simulink library "controllerComponents"  (R2017b)
settings: Solver=VariableStepAuto  StartTime=0.0  StopTime=10.0  RelTol=1e-3
undefined symbols (not defined in the file): ctrl, env, plant
libraries: controllerComponents x14, simulink x3, lowLevel x3, vrlib x1, dspstat3 x1, dspsigops x1
settings Model: Creator=mitch  LastModifiedBy=mitch

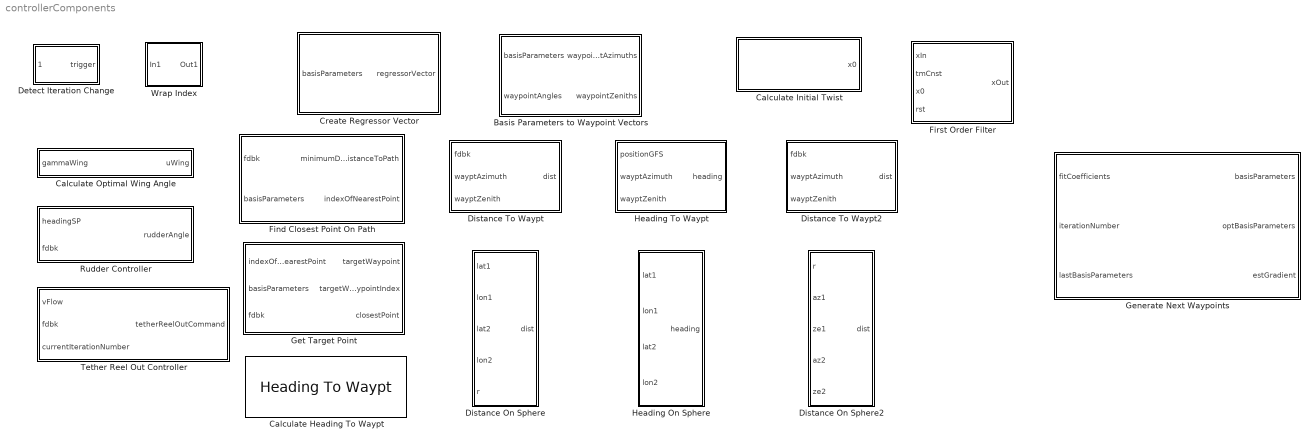
== system controllerComponents ==
  Basis Parameters to Waypoint Vectors : Subsystem
  Calculate Heading To Waypt : controllerComponents/Heading To Waypt
  Calculate Initial Twist : Subsystem
  Calculate Optimal Wing Angle : Subsystem
  Create Regressor Vector : Subsystem
  Detect Iteration Change : Subsystem
  Distance On Sphere : Subsystem
  Distance On Sphere2 : Subsystem
  Distance To Waypt : Subsystem
  Distance To Waypt2 : Subsystem
  Find Closest Point On Path : Subsystem
  First Order Filter : Subsystem
  Generate Next Waypoints : Subsystem
  Get Target Point : Subsystem
  Heading On Sphere : Subsystem
  Heading To Waypt : Subsystem
  Rudder Controller : Subsystem
  Tether Reel Out Controller : Subsystem
  Wrap Index : Subsystem

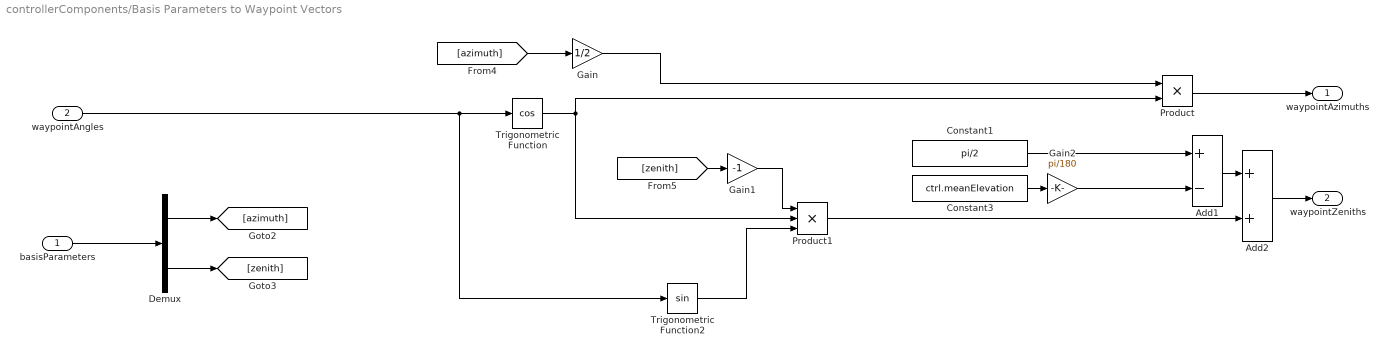
== system controllerComponents/Basis Parameters to Waypoint Vectors ==
  basisParameters : Inport
  waypointAngles : Inport  Port=2
  Add1 : Sum  Inputs=+-
  Add2 : Sum
  Constant1 : Constant  Value=pi/2
  Constant3 : Constant  Value=ctrl.meanElevation
  Demux : Demux  Outputs=2
  Gain : Gain  Gain=1/2
  Gain1 : Gain  Gain=-1
  Gain2 : Gain  Gain=pi/180
  Product : Product
  Product1 : Product  Inputs=3
  Trigonometric Function : Trigonometry  Operator=cos
  Trigonometric Function2 : Trigonometry
  waypointAzimuths : Outport
  waypointZeniths : Outport  Port=2
  wires:
  Gain/1 -> Product/1
  Product1/1 -> Add2/2
  Trigonometric Function2/1 -> Product1/3
  [azimuth] -> Gain/1
  waypointAngles/1 -> Trigonometric Function2/1, Trigonometric Function/1
  basisParameters/1 -> Demux/1
  Demux/1 -> [azimuth]
  [zenith] -> Gain1/1
  Gain1/1 -> Product1/1
  Demux/2 -> [zenith]
  Trigonometric Function/1 -> Product1/2, Product/2
  Constant3/1 -> Gain2/1
  Product/1 -> waypointAzimuths/1
  Add2/1 -> waypointZeniths/1
  Add1/1 -> Add2/1
  Gain2/1 -> Add1/2
  Constant1/1 -> Add1/1

== system controllerComponents/Calculate Initial Twist ==
  Basis Parameters to Waypoint Vectors : controllerComponents/Basis Parameters to Waypoint Vectors
  Constant : Constant  Value=[ctrl.width ctrl.height]
  Constant1 : Constant  Value=ctrl.waypointAngles
  Constant2 : Constant  Value=plant.initialRadius
  Constant3 : Constant  Value=plant.initialAzimuth
  Constant4 : Constant  Value=plant.initialZenith
  Constant5 : Constant  Value=ctrl.lookAheadIndexOffset
  Gain : Gain  Gain=pi/180
  Gain1 : Gain  Gain=pi/180
  Gain2 : Gain  Gain=pi/180
  Heading To Waypt : controllerComponents/Heading To Waypt
  Selector : Selector  InputPortWidth=length(ctrl.waypointAngles)  IndexOptions=Index vector (port)  Indices=2  OutputSizes=1
  Vector Concatenate : Concatenate  NumInputs=3
  x0 : Outport
  wires:
  Gain/1 -> Basis Parameters to Waypoint Vectors/1
  Constant/1 -> Gain/1
  Constant1/1 -> Selector/1
  Selector/1 -> Basis Parameters to Waypoint Vectors/2  "initialWaypointAngle"
  Basis Parameters to Waypoint Vectors/2 -> Heading To Waypt/3  "initialTargetZenith"
  Basis Parameters to Waypoint Vectors/1 -> Heading To Waypt/2  "initialTargetAzimuth"
  Vector Concatenate/1 -> Heading To Waypt/1
  Constant2/1 -> Vector Concatenate/1
  Constant3/1 -> Gain1/1
  Constant4/1 -> Gain2/1
  Gain1/1 -> Vector Concatenate/2
  Gain2/1 -> Vector Concatenate/3
  Heading To Waypt/1 -> x0/1  "initialHeading"
  Constant5/1 -> Selector/2

== system controllerComponents/Calculate Optimal Wing Angle ==
  gammaWing : Inport  Unit=rad
  Add1 : Sum  Inputs=+--
  Add3 : Sum  Inputs=-+
  Add4 : Sum  Inputs=-+
  Constant1 : Constant  Value=plant.wingTable.kl1/(2*plant.wingTable.kd2)
  Constant2 : Constant  Value=plant.wingTable.kd1/(2*plant.wingTable.kd2)
  Constant5 : Constant  Value=max(plant.wingTable.alpha)
  Constant6 : Constant  Value=min(plant.wingTable.alpha)
  Product : Product
  Saturation Dynamic : simulink/Discontinuities/Saturation Dynamic  OutMin=[]  OutMax=[]  OutDataTypeStr=Inherit: Same as second input  OutDataType=fixdt(1, 16)  OutScaling=2^-10  DoSatur=off
  Trigonometric Function : Trigonometry  Operator=tan
  uWing : Outport  Unit=rad
  wires:
  Trigonometric Function/1 -> Product/2
  Product/1 -> Add1/1
  Constant1/1 -> Product/1
  gammaWing/1 -> [gammaWing]
  [gammaWing] -> Add1/2, Trigonometric Function/1
  Add1/1 -> Saturation Dynamic/2  "wingAngleCmdPreSat"
  Saturation Dynamic/1 -> uWing/1
  [gammaWing] -> Add3/1
  Constant5/1 -> Add3/2
  Add3/1 -> Saturation Dynamic/1
  Constant6/1 -> Add4/2
  [gammaWing] -> Add4/1
  Add4/1 -> Saturation Dynamic/3
  Constant2/1 -> Add1/3

== system controllerComponents/Create Regressor Vector ==
  basisParameters : Inport  PortDimensions=2
  Constant2 : Constant
  Demux : Demux  Outputs=2
  Mux : Mux  Inputs=5
  Product : Product
  Product1 : Product
  regressorVector : Outport  PortDimensions=5
  wires:
  Demux/2 -> Product/2, Product/1, Mux/4
  Demux/1 -> Product1/2, Product1/1, Mux/2
  Mux/1 -> regressorVector/1
  Product/1 -> Mux/5
  Constant2/1 -> Mux/1
  Product1/1 -> Mux/3
  basisParameters/1 -> Demux/1

== system controllerComponents/Detect Iteration Change ==
  wyptIdx : Inport
  Add1 : Sum  Inputs=+-
  Compare To Constant : simulink/Logic and Bit Operations/Compare To Constant  relop===  const=-ctrl.num  OutDataTypeStr=boolean
  Delay1 : Delay  DelayLength=1  InitialCondition=0
  trigger : Outport
  wires:
  Add1/1 -> Compare To Constant/1
  wyptIdx/1 -> Delay1/1, Add1/1
  Compare To Constant/1 -> trigger/1
  Delay1/1 -> Add1/2

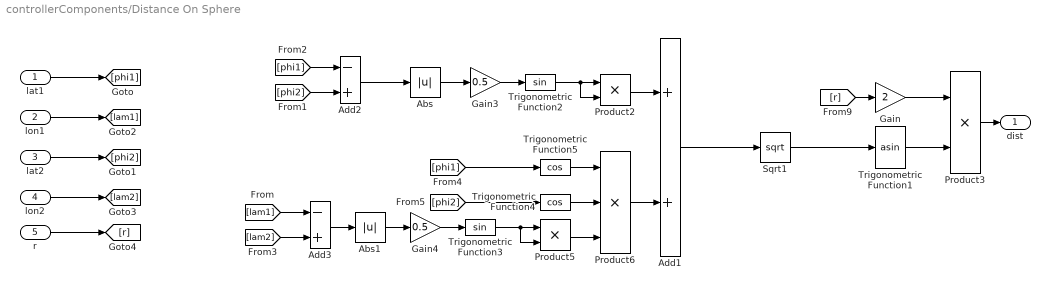
== system controllerComponents/Distance On Sphere ==
  lat1 : Inport
  lon1 : Inport  Port=2
  lat2 : Inport  Port=3
  lon2 : Inport  Port=4
  r : Inport  Port=5
  Abs : Abs
  Abs1 : Abs
  Add1 : Sum
  Add2 : Sum  Inputs=-+
  Add3 : Sum  Inputs=-+
  Gain : Gain  Gain=2
  Gain3 : Gain  Gain=0.5
  Gain4 : Gain  Gain=0.5
  Product2 : Product
  Product3 : Product
  Product5 : Product
  Product6 : Product  Inputs=3
  Sqrt1 : Sqrt  SaturateOnIntegerOverflow=on
  Trigonometric Function1 : Trigonometry  Operator=asin
  Trigonometric Function2 : Trigonometry
  Trigonometric Function3 : Trigonometry
  Trigonometric Function4 : Trigonometry  Operator=cos
  Trigonometric Function5 : Trigonometry  Operator=cos
  dist : Outport
  wires:
  Trigonometric Function1/1 -> Product3/2
  Abs1/1 -> Gain4/1
  Abs/1 -> Gain3/1
  Sqrt1/1 -> Trigonometric Function1/1
  Product6/1 -> Add1/2
  [phi2] -> Trigonometric Function4/1
  [phi1] -> Trigonometric Function5/1
  Trigonometric Function5/1 -> Product6/1
  Trigonometric Function4/1 -> Product6/2
  Product5/1 -> Product6/3
  [lam2] -> Add3/2
  [lam1] -> Add3/1
  Add3/1 -> Abs1/1
  Gain4/1 -> Trigonometric Function3/1
  Trigonometric Function3/1 -> Product5/2, Product5/1
  [phi2] -> Add2/2
  [phi1] -> Add2/1
  Product2/1 -> Add1/1
  Trigonometric Function2/1 -> Product2/2, Product2/1
  Gain3/1 -> Trigonometric Function2/1
  Add2/1 -> Abs/1
  lon1/1 -> [lam1]
  lat1/1 -> [phi1]
  lat2/1 -> [phi2]
  lon2/1 -> [lam2]
  r/1 -> [r]
  Product3/1 -> dist/1
  [r] -> Gain/1
  Gain/1 -> Product3/1
  Add1/1 -> Sqrt1/1

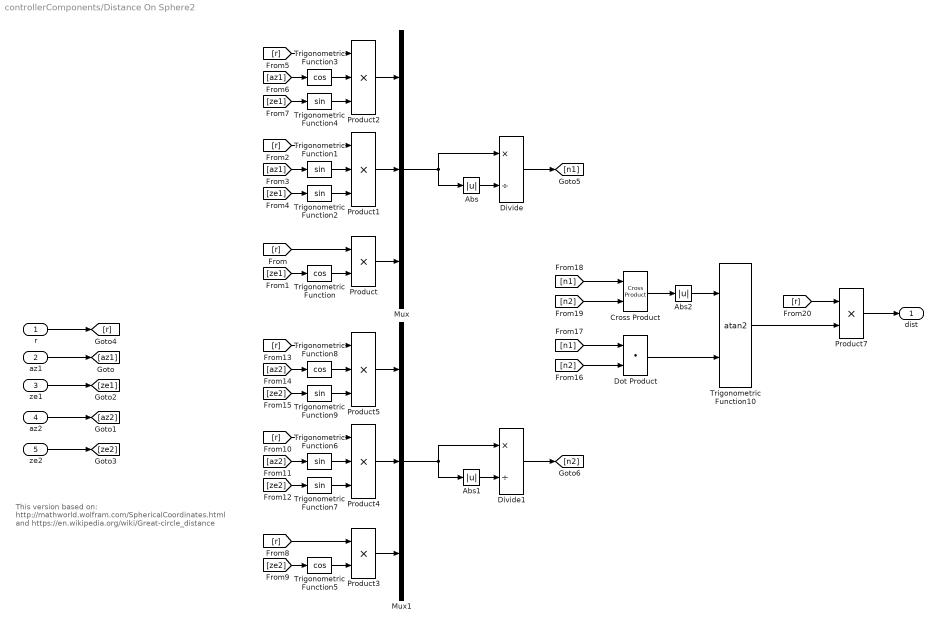
== system controllerComponents/Distance On Sphere2 ==
  note: This version based on:
      | http://mathworld.wolfram.com/SphericalCoordinates.html
      | and
      | https://en.wikipedia.org/wiki/Great-circle_distance
  r : Inport
  az1 : Inport  Port=2
  ze1 : Inport  Port=3
  az2 : Inport  Port=4
  ze2 : Inport  Port=5
  Abs : Abs
  Abs1 : Abs
  Abs2 : Abs
  Cross Product : vrlib/Utilities/Cross Product
      settings: SourceProductBaseCode=VR
  Divide : Product  Inputs=*/
  Divide1 : Product  Inputs=*/
  Dot Product : DotProduct  InputSameDT=on  OutDataTypeStr=Inherit: Inherit via internal rule
  Mux : Mux  Inputs=3
  Mux1 : Mux  Inputs=3
  Product : Product
  Product{1..2,4..5} (4 alike) : Product  Inputs=3
  Product3 : Product
  Product7 : Product
  Trigonometric Function{,3,5,8} (4 alike) : Trigonometry  Operator=cos
  Trigonometric Function{1..2,4,6..7,9} (6 alike) : Trigonometry
  Trigonometric Function10 : Trigonometry  Operator=atan2
  dist : Outport
  wires:
  ze1/1 -> [ze1]
  az1/1 -> [az1]
  az2/1 -> [az2]
  ze2/1 -> [ze2]
  r/1 -> [r]
  Trigonometric Function/1 -> Product/2
  [r] -> Product/1
  [ze1] -> Trigonometric Function/1
  Trigonometric Function2/1 -> Product1/3
  Trigonometric Function1/1 -> Product1/2
  [r] -> Product1/1
  [az1] -> Trigonometric Function1/1
  [ze1] -> Trigonometric Function2/1
  [r] -> Product2/1
  [ze1] -> Trigonometric Function4/1
  [az1] -> Trigonometric Function3/1
  Trigonometric Function3/1 -> Product2/2
  Trigonometric Function4/1 -> Product2/3
  Product/1 -> Mux/3
  Product1/1 -> Mux/2
  Product2/1 -> Mux/1
  Product4/1 -> Mux1/2
  Product5/1 -> Mux1/1
  [r] -> Product4/1
  Trigonometric Function8/1 -> Product5/2
  [az2] -> Trigonometric Function8/1
  Trigonometric Function9/1 -> Product5/3
  [ze2] -> Trigonometric Function7/1
  [ze2] -> Trigonometric Function9/1
  Product3/1 -> Mux1/3
  Trigonometric Function5/1 -> Product3/2
  [r] -> Product5/1
  Trigonometric Function6/1 -> Product4/2
  Trigonometric Function7/1 -> Product4/3
  [az2] -> Trigonometric Function6/1
  [ze2] -> Trigonometric Function5/1
  [r] -> Product3/1
  Abs/1 -> Divide/2
  Mux/1 -> Abs/1, Divide/1
  Abs1/1 -> Divide1/2
  Mux1/1 -> Divide1/1, Abs1/1
  Divide/1 -> [n1]
  Divide1/1 -> [n2]
  [n2] -> Dot Product/2
  [n1] -> Dot Product/1
  [n1] -> Cross Product/1
  [n2] -> Cross Product/2
  Cross Product/1 -> Abs2/1
  Dot Product/1 -> Trigonometric Function10/2
  Abs2/1 -> Trigonometric Function10/1
  Trigonometric Function10/1 -> Product7/2
  [r] -> Product7/1
  Product7/1 -> dist/1

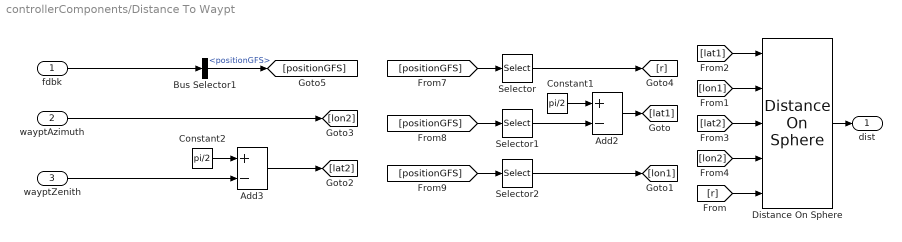
== system controllerComponents/Distance To Waypt ==
  fdbk : Inport
  wayptAzimuth : Inport  Port=2
  wayptZenith : Inport  Port=3
  Add2 : Sum  Inputs=+-
  Add3 : Sum  Inputs=+-
  Bus Selector1 : BusSelector  OutputSignals=positionGFS
  Constant1 : Constant  Value=pi/2
  Constant2 : Constant  Value=pi/2
  Distance On Sphere : controllerComponents/Distance On Sphere
  Selector : Selector  InputPortWidth=3  IndexOptions=Index vector (dialog)  Indices=1  OutputSizes=1
  Selector1 : Selector  InputPortWidth=3  IndexOptions=Index vector (dialog)  Indices=3  OutputSizes=1
  Selector2 : Selector  InputPortWidth=3  IndexOptions=Index vector (dialog)  Indices=2  OutputSizes=1
  dist : Outport
  wires:
  wayptAzimuth/1 -> [lon2]
  fdbk/1 -> Bus Selector1/1
  Bus Selector1/1 -> [positionGFS]  "<positionGFS>"
  [positionGFS] -> Selector/1
  Selector/1 -> [r]
  [positionGFS] -> Selector1/1
  Constant1/1 -> Add2/1
  Add2/1 -> [lat1]
  Selector1/1 -> Add2/2
  [positionGFS] -> Selector2/1
  Selector2/1 -> [lon1]
  Constant2/1 -> Add3/1
  wayptZenith/1 -> Add3/2
  Add3/1 -> [lat2]
  Distance On Sphere/1 -> dist/1
  [r] -> Distance On Sphere/5
  [lon1] -> Distance On Sphere/2
  [lat1] -> Distance On Sphere/1
  [lat2] -> Distance On Sphere/3
  [lon2] -> Distance On Sphere/4

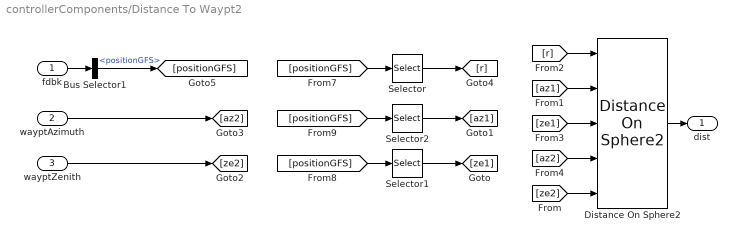
== system controllerComponents/Distance To Waypt2 ==
  fdbk : Inport
  wayptAzimuth : Inport  Port=2
  wayptZenith : Inport  Port=3
  Bus Selector1 : BusSelector  OutputSignals=positionGFS
  Distance On Sphere2 : controllerComponents/Distance On Sphere2
  Selector : Selector  InputPortWidth=3  IndexOptions=Index vector (dialog)  Indices=1  OutputSizes=1
  Selector1 : Selector  InputPortWidth=3  IndexOptions=Index vector (dialog)  Indices=3  OutputSizes=1
  Selector2 : Selector  InputPortWidth=3  IndexOptions=Index vector (dialog)  Indices=2  OutputSizes=1
  dist : Outport
  wires:
  wayptAzimuth/1 -> [az2]
  fdbk/1 -> Bus Selector1/1
  Bus Selector1/1 -> [positionGFS]  "<positionGFS>"
  [positionGFS] -> Selector/1
  Selector/1 -> [r]
  [positionGFS] -> Selector1/1
  [positionGFS] -> Selector2/1
  Selector2/1 -> [az1]
  Distance On Sphere2/1 -> dist/1
  [ze2] -> Distance On Sphere2/5
  [az1] -> Distance On Sphere2/2
  [r] -> Distance On Sphere2/1
  [ze1] -> Distance On Sphere2/3
  [az2] -> Distance On Sphere2/4
  wayptZenith/1 -> [ze2]
  Selector1/1 -> [ze1]

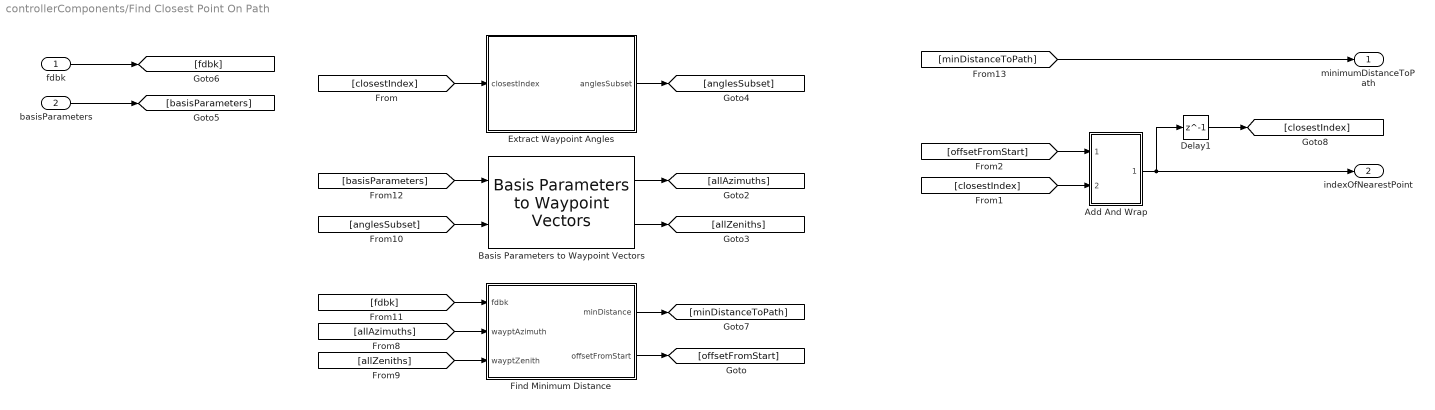
== system controllerComponents/Find Closest Point On Path ==
  fdbk : Inport
  basisParameters : Inport  Port=2
  Add And Wrap : Subsystem
  Basis Parameters to Waypoint Vectors : controllerComponents/Basis Parameters to Waypoint Vectors
  Delay1 : Delay  DelayLength=1  InitialCondition=1
  Extract Waypoint Angles : Subsystem
  Find Minimum Distance : Subsystem
  minimumDistanceToPath : Outport
  indexOfNearestPoint : Outport  Port=2
  wires:
  [closestIndex] -> Extract Waypoint Angles/1(closestIndex)
  Basis Parameters to Waypoint Vectors/2 -> [allZeniths]
  Basis Parameters to Waypoint Vectors/1 -> [allAzimuths]
  Extract Waypoint Angles/1(anglesSubset) -> [anglesSubset]
  [anglesSubset] -> Basis Parameters to Waypoint Vectors/2
  basisParameters/1 -> [basisParameters]
  fdbk/1 -> [fdbk]
  [basisParameters] -> Basis Parameters to Waypoint Vectors/1
  [minDistanceToPath] -> minimumDistanceToPath/1
  [fdbk] -> Find Minimum Distance/1(fdbk)
  [allAzimuths] -> Find Minimum Distance/2(wayptAzimuth)
  [allZeniths] -> Find Minimum Distance/3(wayptZenith)
  Find Minimum Distance/1(minDistance) -> [minDistanceToPath]
  Find Minimum Distance/2(offsetFromStart) -> [offsetFromStart]
  [offsetFromStart] -> Add And Wrap/1(offset)
  [closestIndex] -> Add And Wrap/2(startIndex)
  Add And Wrap/1(Out1) -> Delay1/1, indexOfNearestPoint/1
  Delay1/1 -> [closestIndex]

== system controllerComponents/First Order Filter ==
  xIn : Inport
  tmCnst : Inport  Port=2
  x0 : Inport  Port=3
  rst : Inport  Port=4
  Add : Sum  Inputs=+-
  Divide : Product  Inputs=*/
  Integrator : Integrator  ExternalReset=rising  InitialConditionSource=external
  xOut : Outport
  wires:
  x0/1 -> Integrator/3
  rst/1 -> Integrator/2
  Integrator/1 -> Add/2, xOut/1
  Divide/1 -> Integrator/1
  Add/1 -> Divide/1
  tmCnst/1 -> Divide/2
  xIn/1 -> Add/1

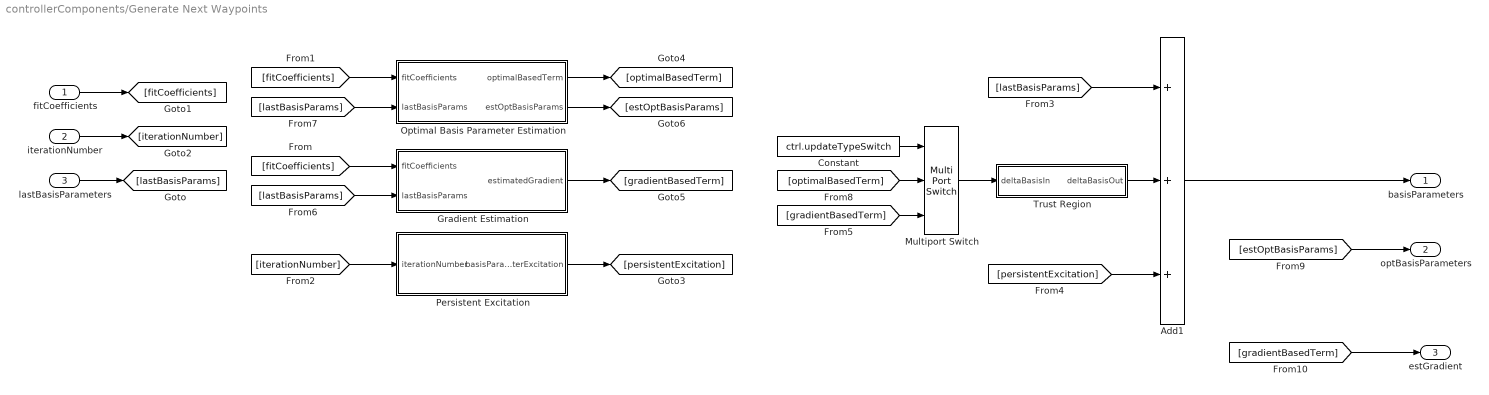
== system controllerComponents/Generate Next Waypoints ==
  fitCoefficients : Inport  PortDimensions=5
  iterationNumber : Inport  Port=2
  lastBasisParameters : Inport  Port=3
  Add1 : Sum  Inputs=+++
  Constant : Constant  Value=ctrl.updateTypeSwitch
  Gradient Estimation : Subsystem
  Multiport Switch : MultiPortSwitch  Inputs=2
  Optimal Basis Parameter Estimation : Subsystem
  Persistent Excitation : Subsystem
  Trust Region : Subsystem
  basisParameters : Outport
  optBasisParameters : Outport  Port=2
  estGradient : Outport  Port=3
  wires:
  [persistentExcitation] -> Add1/3
  Trust Region/1(deltaBasisOut) -> Add1/2
  Constant/1 -> Multiport Switch/1
  [gradientBasedTerm] -> Multiport Switch/3
  [optimalBasedTerm] -> Multiport Switch/2
  [estOptBasisParams] -> optBasisParameters/1
  Optimal Basis Parameter Estimation/2(estOptBasisParams) -> [estOptBasisParams]
  [lastBasisParams] -> Optimal Basis Parameter Estimation/2(lastBasisParams)
  [lastBasisParams] -> Gradient Estimation/2(lastBasisParams)
  Optimal Basis Parameter Estimation/1(optimalBasedTerm) -> [optimalBasedTerm]
  Gradient Estimation/1(estimatedGradient) -> [gradientBasedTerm]
  Persistent Excitation/1(basisParameterExcitation) -> [persistentExcitation]
  [iterationNumber] -> Persistent Excitation/1(iterationNumber)
  iterationNumber/1 -> [iterationNumber]
  [fitCoefficients] -> Optimal Basis Parameter Estimation/1(fitCoefficients)
  fitCoefficients/1 -> [fitCoefficients]
  lastBasisParameters/1 -> [lastBasisParams]
  Multiport Switch/1 -> Trust Region/1(deltaBasisIn)
  Add1/1 -> basisParameters/1
  [lastBasisParams] -> Add1/1
  [fitCoefficients] -> Gradient Estimation/1(fitCoefficients)
  [gradientBasedTerm] -> estGradient/1

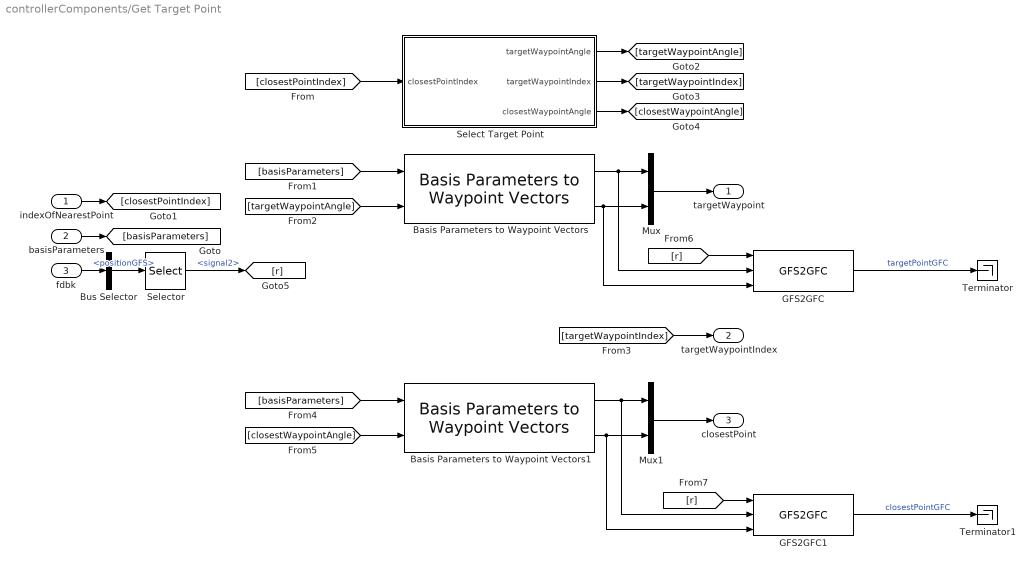
== system controllerComponents/Get Target Point ==
  indexOfNearestPoint : Inport
  basisParameters : Inport  Port=2
  fdbk : Inport  Port=3  OutDataTypeStr=Bus: busPlantFeedback
  Basis Parameters to Waypoint Vectors : controllerComponents/Basis Parameters to Waypoint Vectors
  Basis Parameters to Waypoint Vectors1 : controllerComponents/Basis Parameters to Waypoint Vectors
  Bus Selector : BusSelector  OutputSignals=positionGFS
  GFS2GFC : lowLevel/GFS2GFC
  GFS2GFC1 : lowLevel/GFS2GFC
  Mux : Mux  Inputs=2
  Mux1 : Mux  Inputs=2
  Select Target Point : Subsystem
  Selector : Selector  InputPortWidth=3  IndexOptions=Index vector (dialog)  Indices=1  OutputSizes=1
  Terminator : Terminator
  Terminator1 : Terminator
  targetWaypoint : Outport
  targetWaypointIndex : Outport  Port=2
  closestPoint : Outport  Port=3
  wires:
  Basis Parameters to Waypoint Vectors/1 -> GFS2GFC/2, Mux/1
  Basis Parameters to Waypoint Vectors/2 -> GFS2GFC/3, Mux/2
  basisParameters/1 -> [basisParameters]
  indexOfNearestPoint/1 -> [closestPointIndex]
  [closestPointIndex] -> Select Target Point/1(closestPointIndex)
  [basisParameters] -> Basis Parameters to Waypoint Vectors/1
  Select Target Point/1(targetWaypointAngle) -> [targetWaypointAngle]
  Mux/1 -> targetWaypoint/1
  [targetWaypointAngle] -> Basis Parameters to Waypoint Vectors/2
  Select Target Point/2(targetWaypointIndex) -> [targetWaypointIndex]
  Select Target Point/3(closestWaypointAngle) -> [closestWaypointAngle]
  [targetWaypointIndex] -> targetWaypointIndex/1
  Basis Parameters to Waypoint Vectors1/2 -> GFS2GFC1/3, Mux1/2
  Basis Parameters to Waypoint Vectors1/1 -> GFS2GFC1/2, Mux1/1
  [basisParameters] -> Basis Parameters to Waypoint Vectors1/1
  Mux1/1 -> closestPoint/1
  [closestWaypointAngle] -> Basis Parameters to Waypoint Vectors1/2
  GFS2GFC/1 -> Terminator/1  "targetPointGFC"
  GFS2GFC1/1 -> Terminator1/1  "closestPointGFC"
  fdbk/1 -> Bus Selector/1
  Selector/1 -> [r]  "<signal2>"
  Bus Selector/1 -> Selector/1  "<positionGFS>"
  [r] -> GFS2GFC/1
  [r] -> GFS2GFC1/1

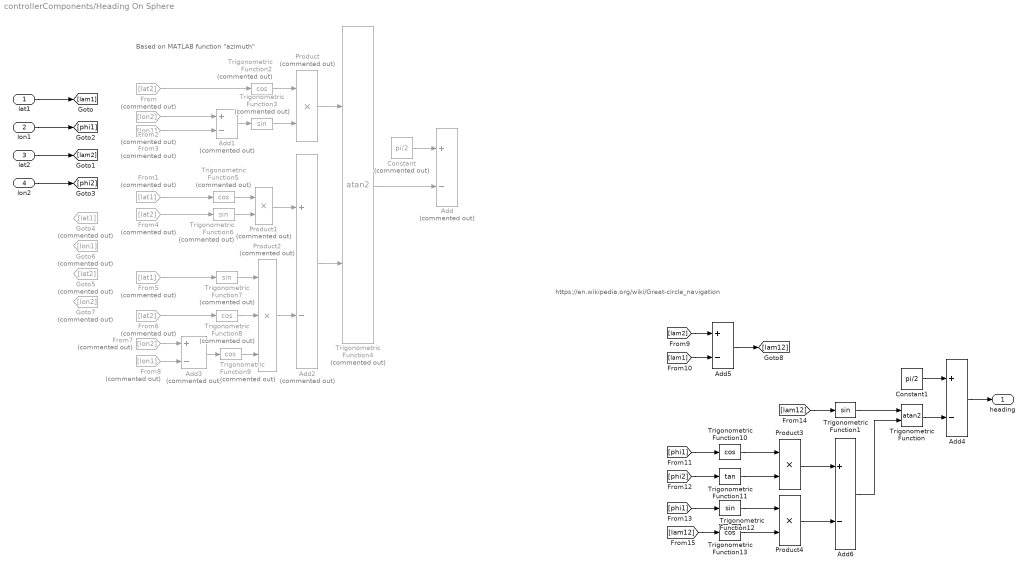
== system controllerComponents/Heading On Sphere ==
  note: Based on MATLAB function "azimuth"
  note: https://en.wikipedia.org/wiki/Great-circle_navigation
  lat1 : Inport
  lon1 : Inport  Port=2
  lat2 : Inport  Port=3
  lon2 : Inport  Port=4
  Add{,1..3} (4 alike) : Sum  Commented=on  Inputs=+-
  Add4 : Sum  Inputs=+-
  Add5 : Sum  Inputs=+-
  Add6 : Sum  Inputs=+-
  Constant : Constant  Commented=on  Value=pi/2
  Constant1 : Constant  Value=pi/2
  From : From  Commented=on  GotoTag=lat2
  From1 : From  Commented=on  GotoTag=lat1
  From2 : From  Commented=on  GotoTag=lon2
  From3 : From  Commented=on  GotoTag=lon1
  From4 : From  Commented=on  GotoTag=lat2
  From5 : From  Commented=on  GotoTag=lat1
  From6 : From  Commented=on  GotoTag=lat2
  From7 : From  Commented=on  GotoTag=lon2
  From8 : From  Commented=on  GotoTag=lon1
  Goto4 : Goto  Commented=on  GotoTag=lat1
  Goto5 : Goto  Commented=on  GotoTag=lat2
  Goto6 : Goto  Commented=on  GotoTag=lon1
  Goto7 : Goto  Commented=on  GotoTag=lon2
  Product : Product  Commented=on
  Product1 : Product  Commented=on
  Product2 : Product  Commented=on  Inputs=3
  Product3 : Product
  Product4 : Product
  Trigonometric Function : Trigonometry  Operator=atan2
  Trigonometric Function1 : Trigonometry
  Trigonometric Function10 : Trigonometry  Operator=cos
  Trigonometric Function11 : Trigonometry  Operator=tan
  Trigonometric Function12 : Trigonometry
  Trigonometric Function13 : Trigonometry  Operator=cos
  Trigonometric Function{2,5,8..9} (4 alike) : Trigonometry  Commented=on  Operator=cos
  Trigonometric Function3 : Trigonometry  Commented=on
  Trigonometric Function4 : Trigonometry  Commented=on  Operator=atan2
  Trigonometric Function6 : Trigonometry  Commented=on
  Trigonometric Function7 : Trigonometry  Commented=on
  heading : Outport
  wires:
  From2/1 -> Add1/1
  Trigonometric Function4/1 -> Add/2
  From4/1 -> Trigonometric Function6/1
  Trigonometric Function3/1 -> Product/2
  Trigonometric Function2/1 -> Product/1
  Add1/1 -> Trigonometric Function3/1
  Product1/1 -> Add2/1
  From1/1 -> Trigonometric Function5/1
  Add2/1 -> Trigonometric Function4/2
  From8/1 -> Add3/2
  From/1 -> Trigonometric Function2/1
  Add3/1 -> Trigonometric Function9/1
  From6/1 -> Trigonometric Function8/1
  Trigonometric Function5/1 -> Product1/1
  Trigonometric Function7/1 -> Product2/1
  From7/1 -> Add3/1
  Product/1 -> Trigonometric Function4/1
  Trigonometric Function9/1 -> Product2/3
  From3/1 -> Add1/2
  Trigonometric Function6/1 -> Product1/2
  Product2/1 -> Add2/2
  From5/1 -> Trigonometric Function7/1
  Trigonometric Function8/1 -> Product2/2
  lon2/1 -> [phi2]
  lat2/1 -> [lam2]
  lat1/1 -> [lam1]
  lon1/1 -> [phi1]
  Constant/1 -> Add/1
  Trigonometric Function10/1 -> Product3/1
  Trigonometric Function13/1 -> Product4/2
  Add5/1 -> [lam12]
  [lam1] -> Add5/2
  [phi2] -> Trigonometric Function11/1
  [phi1] -> Trigonometric Function10/1
  [lam12] -> Trigonometric Function13/1
  [lam12] -> Trigonometric Function1/1
  [phi1] -> Trigonometric Function12/1
  Add6/1 -> Trigonometric Function/2
  Trigonometric Function1/1 -> Trigonometric Function/1
  Product4/1 -> Add6/2
  Trigonometric Function12/1 -> Product4/1
  Constant1/1 -> Add4/1
  [lam2] -> Add5/1
  Add4/1 -> heading/1
  Product3/1 -> Add6/1
  Trigonometric Function/1 -> Add4/2
  Trigonometric Function11/1 -> Product3/2

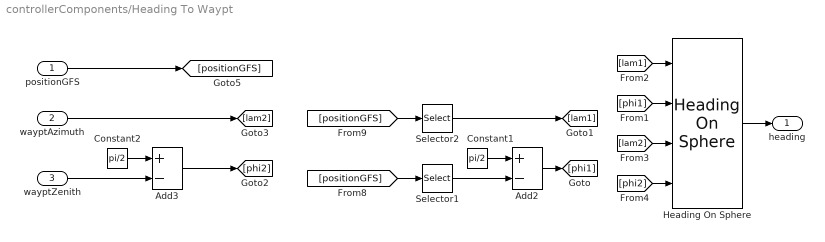
== system controllerComponents/Heading To Waypt ==
  positionGFS : Inport
  wayptAzimuth : Inport  Port=2
  wayptZenith : Inport  Port=3
  Add2 : Sum  Inputs=+-
  Add3 : Sum  Inputs=+-
  Constant1 : Constant  Value=pi/2
  Constant2 : Constant  Value=pi/2
  Heading On Sphere : controllerComponents/Heading  On Sphere
  Selector1 : Selector  InputPortWidth=3  IndexOptions=Index vector (dialog)  Indices=3  OutputSizes=1
  Selector2 : Selector  InputPortWidth=3  IndexOptions=Index vector (dialog)  Indices=2  OutputSizes=1
  heading : Outport
  wires:
  [phi2] -> Heading On Sphere/4
  [lam2] -> Heading On Sphere/3
  [lam1] -> Heading On Sphere/1
  [phi1] -> Heading On Sphere/2
  Heading On Sphere/1 -> heading/1
  Add3/1 -> [phi2]
  wayptZenith/1 -> Add3/2
  Constant2/1 -> Add3/1
  Selector2/1 -> [lam1]
  [positionGFS] -> Selector2/1
  Selector1/1 -> Add2/2
  Add2/1 -> [phi1]
  Constant1/1 -> Add2/1
  [positionGFS] -> Selector1/1
  positionGFS/1 -> [positionGFS]
  wayptAzimuth/1 -> [lam2]

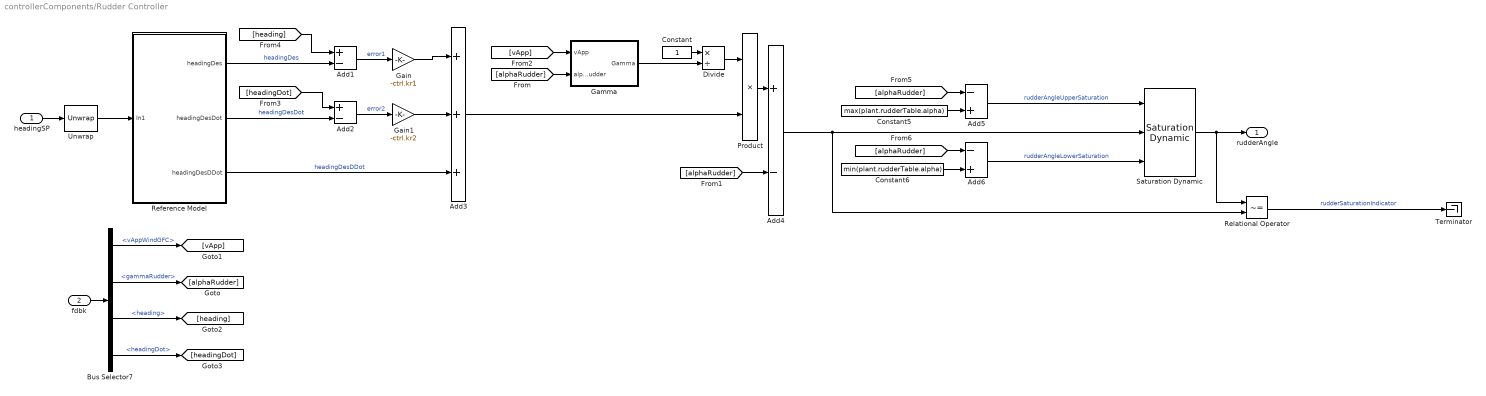
== system controllerComponents/Rudder Controller ==
  headingSP : Inport  Unit=rad
  fdbk : Inport  Port=2  OutDataTypeStr=Bus: busPlantFeedback
  Add1 : Sum  Inputs=+-
  Add2 : Sum  Inputs=+-
  Add3 : Sum  Inputs=+++
  Add4 : Sum  Inputs=+-
  Add5 : Sum  Inputs=-+
  Add6 : Sum  Inputs=-+
  Bus Selector7 : BusSelector  OutputSignals=vAppWindGFC,gammaRudder,heading,headingDot
  Constant : Constant
  Constant5 : Constant  Value=max(plant.rudderTable.alpha)
  Constant6 : Constant  Value=min(plant.rudderTable.alpha)
  Divide : Product  Inputs=*/
  Gain : Gain  Gain=-ctrl.kr1
  Gain1 : Gain  Gain=-ctrl.kr2
  Gamma : Subsystem
  Product : Product
  Reference Model : Subsystem
  Relational Operator : RelationalOperator  Operator=~=  OutDataTypeStr=boolean  RndMeth=Simplest
  Saturation Dynamic : simulink/Discontinuities/Saturation Dynamic  OutMin=[]  OutMax=[]  OutDataTypeStr=Inherit: Same as second input  OutDataType=fixdt(1, 16)  OutScaling=2^-10  DoSatur=off
  Terminator : Terminator
  Unwrap : dspsigops/Unwrap  tol=pi  InputProcessing=Columns as channels (frame based)  running=off
  rudderAngle : Outport  Unit=rad
  wires:
  [vApp] -> Gamma/1(vApp)
  [alphaRudder] -> Gamma/2(alphaRudder)
  [alphaRudder] -> Add4/2
  Product/1 -> Add4/1
  Gamma/1(Gamma) -> Divide/2
  Divide/1 -> Product/1
  Constant/1 -> Divide/1
  Add2/1 -> Gain1/1  "error2"
  Add1/1 -> Gain/1  "error1"
  Reference Model/1(headingDes) -> Add1/2  "headingDes"
  Reference Model/2(headingDesDot) -> Add2/2  "headingDesDot"
  [heading] -> Add1/1
  Gain1/1 -> Add3/2
  [headingDot] -> Add2/1
  Reference Model/3(headingDesDDot) -> Add3/3  "headingDesDDot"
  Gain/1 -> Add3/1
  headingSP/1 -> Unwrap/1
  Add3/1 -> Product/2
  fdbk/1 -> Bus Selector7/1
  Bus Selector7/4 -> [headingDot]  "<headingDot>"
  Bus Selector7/3 -> [heading]  "<heading>"
  Bus Selector7/2 -> [alphaRudder]  "<gammaRudder>"
  Bus Selector7/1 -> [vApp]  "<vAppWindGFC>"
  [alphaRudder] -> Add6/1
  Add6/1 -> Saturation Dynamic/3  "rudderAngleLowerSaturation"
  Constant6/1 -> Add6/2
  Constant5/1 -> Add5/2
  Add5/1 -> Saturation Dynamic/1  "rudderAngleUpperSaturation"
  [alphaRudder] -> Add5/1
  Saturation Dynamic/1 -> Relational Operator/1, rudderAngle/1
  Add4/1 -> Relational Operator/2, Saturation Dynamic/2
  Unwrap/1 -> Reference Model/1(In1)
  Relational Operator/1 -> Terminator/1  "rudderSaturationIndicator"

== system controllerComponents/Tether Reel Out Controller ==
  vFlow : Inport
  fdbk : Inport  Port=2  OutDataTypeStr=Bus: busPlantFeedback
  currentIterationNumber : Inport  Port=3
  Bus Selector : BusSelector  OutputSignals=positionGFS
  Constant : Constant  Value=0
  Constant1 : Constant  Value=ctrl.numSettlingLaps
  Constant2 : Constant  Value=0
  Constant3 : Constant  Value=ctrl.tetherReelOutFilterTimeConstant
  Constant4 : Constant  Value=plant.initialRadiusRate
  Divide : Product  Inputs=*/
  Dot Product : DotProduct  InputSameDT=on  OutDataTypeStr=Inherit: Inherit via internal rule
  First Order Filter : controllerComponents/First Order Filter
  Gain : Gain  Gain=3
  Multiport Switch : MultiPortSwitch  DataPortOrder=Zero-based contiguous  Inputs=2
  Relational Operator : RelationalOperator  Operator=>  OutDataTypeStr=boolean  RndMeth=Simplest
  Selector : Selector  InputPortWidth=3  IndexOptions=Index vector (dialog)  Indices=3  OutputSizes=1
  Sqrt : Sqrt  SaturateOnIntegerOverflow=on
  Trigonometric Function : Trigonometry
  tetherReelOutCommand : Outport
  wires:
  currentIterationNumber/1 -> Relational Operator/1
  Constant1/1 -> Relational Operator/2
  Relational Operator/1 -> Multiport Switch/1
  Constant/1 -> Multiport Switch/2
  fdbk/1 -> Bus Selector/1
  Bus Selector/1 -> Selector/1  "<positionGFS>"
  Selector/1 -> Trigonometric Function/1
  vFlow/1 -> Dot Product/1, Dot Product/2
  Dot Product/1 -> Sqrt/1
  Multiport Switch/1 -> First Order Filter/1
  First Order Filter/1 -> tetherReelOutCommand/1
  Constant2/1 -> First Order Filter/4
  Constant3/1 -> First Order Filter/2
  Divide/1 -> Multiport Switch/3
  Trigonometric Function/1 -> Gain/1
  Gain/1 -> Divide/2
  Sqrt/1 -> Divide/1
  Constant4/1 -> First Order Filter/3

== system controllerComponents/Wrap Index ==
  In1 : Inport
  Add : Sum
  Constant2 : Constant  Value=length(ctrl.waypointAngles)  SampleTime=-1
  Constant3 : Constant  SampleTime=-1
  Math Function : Math  Operator=mod  SaturateOnIntegerOverflow=on
  Out1 : Outport
  wires:
  Math Function/1 -> Add/2
  Constant2/1 -> Math Function/2
  Constant3/1 -> Add/1
  In1/1 -> Math Function/1
  Add/1 -> Out1/1

== system controllerComponents/Find Closest Point On Path/Add And Wrap ==
  offset : Inport
  startIndex : Inport  Port=2
  Add1 : Sum
  Constant2 : Constant  Value=length(ctrl.waypointAngles)+0.5  SampleTime=-1
  Math Function : Math  Operator=mod  SaturateOnIntegerOverflow=on
  Round : Rounding  Operator=round
  Out1 : Outport
  wires:
  offset/1 -> Add1/1
  startIndex/1 -> Add1/2
  Add1/1 -> Math Function/1
  Constant2/1 -> Math Function/2
  Math Function/1 -> Round/1
  Round/1 -> Out1/1

== system controllerComponents/Find Closest Point On Path/Extract Waypoint Angles ==
  closestIndex : Inport
  Add4 : Sum
  Constant1 : Constant  Value=ctrl.waypointAngles  SampleTime=-1
  Constant2 : Constant  Value=ctrl.localSearchIndexOffsetVector  SampleTime=-1
  Selector : Selector  InputPortWidth=length(ctrl.waypointAngles)  IndexOptions=Index vector (port)  Indices=[1 3]  OutputSizes=1
  Wrap Index : controllerComponents/Wrap Index
  anglesSubset : Outport
  wires:
  Selector/1 -> anglesSubset/1
  Wrap Index/1 -> Selector/2
  Add4/1 -> Wrap Index/1
  Constant2/1 -> Add4/2
  Constant1/1 -> Selector/1
  closestIndex/1 -> Add4/1

== system controllerComponents/Find Closest Point On Path/Find Minimum Distance ==
  fdbk : Inport
  wayptAzimuth : Inport  Port=2
  wayptZenith : Inport  Port=3
  Distance To Waypt : controllerComponents/Distance To Waypt
  Minimum : dspstat3/Minimum  operation=minimum  fcn=Value and Index  indexBase=Zero  operateOver=Entire input  Dimension=1  InputProcessing=Columns as channels (frame based)  reset=None  roiEnable=off  roiType=Rectangles  roiPortion=Entire ROI  roiOutput=Individual statistics for each ROI  roiFlag=off  roundingMode=Floor  overflowMode=off
      settings: SourceProductName=DSP System Toolbox  SourceProductBaseCode=DS
  minDistance : Outport
  offsetFromStart : Outport  Port=2
  wires:
  Distance To Waypt/1 -> Minimum/1  "distances"
  wayptAzimuth/1 -> Distance To Waypt/2
  Minimum/1 -> minDistance/1
  wayptZenith/1 -> Distance To Waypt/3
  fdbk/1 -> Distance To Waypt/1
  Minimum/2 -> offsetFromStart/1  "offsetFromStart"

== system controllerComponents/Generate Next Waypoints/Gradient Estimation ==
  fitCoefficients : Inport  PortDimensions=5
  lastBasisParams : Inport  Port=2  PortDimensions=2
  Add : Sum
  Add1 : Sum
  Demux : Demux  Outputs=5
  Demux1 : Demux  Outputs=2
  Gain : Gain  Gain=2
  Gain2 : Gain  Gain=2
  Mux : Mux  Inputs=2
  Product : Product
  Product1 : Product
  Terminator : Terminator
  estimatedGradient : Outport
  wires:
  Demux/4 -> Add1/1
  Demux/5 -> Gain2/1
  [zenith] -> Product1/1
  Gain2/1 -> Product1/2
  Add1/1 -> Mux/2
  Product1/1 -> Add1/2
  Gain/1 -> Product/2
  [azimuth] -> Product/1
  Product/1 -> Add/2
  Demux1/2 -> [zenith]
  Demux1/1 -> [azimuth]
  lastBasisParams/1 -> Demux1/1
  Demux/3 -> Gain/1
  Demux/2 -> Add/1
  Add/1 -> Mux/1
  Demux/1 -> Terminator/1
  Mux/1 -> estimatedGradient/1
  fitCoefficients/1 -> Demux/1

== system controllerComponents/Generate Next Waypoints/Optimal Basis Parameter Estimation ==
  fitCoefficients : Inport  PortDimensions=5
  lastBasisParams : Inport  Port=2  PortDimensions=2
  Add : Sum  Inputs=+-
  Add1 : Sum  Inputs=-+
  Constant : Constant  Value=ctrl.updateTypeSwitch
  Constant1 : Constant  Value=ctrl.KLearningNewton
  Constant2 : Constant  Value=ctrl.KLearningGradient
  Demux : Demux  Outputs=5
  Demux1 : Demux  Outputs=2
  Divide : Product  Inputs=*/
  Divide1 : Product  Inputs=*/
  Gain : Gain  Gain=-2
  Gain1 : Gain  Gain=-2
  Multiport Switch : MultiPortSwitch  Inputs=2
  Mux1 : Mux  Inputs=2
  Mux2 : Mux  Inputs=2
  Product : Product
  Terminator : Terminator
  optimalBasedTerm : Outport
  estOptBasisParams : Outport  Port=2
  wires:
  Mux2/1 -> estOptBasisParams/1
  Add/1 -> Mux1/1
  Add1/1 -> Mux1/2
  Divide1/1 -> Add1/2, Mux2/2
  Divide/1 -> Add/1, Mux2/1
  Demux1/2 -> Add1/1
  Demux1/1 -> Add/2
  lastBasisParams/1 -> Demux1/1
  Demux/2 -> Divide/1
  Demux/1 -> Terminator/1
  Demux/3 -> Gain/1
  Gain1/1 -> Divide1/2
  Gain/1 -> Divide/2
  Demux/4 -> Divide1/1
  fitCoefficients/1 -> Demux/1
  Demux/5 -> Gain1/1
  Multiport Switch/1 -> Product/1
  Product/1 -> optimalBasedTerm/1
  Mux1/1 -> Product/2
  Constant/1 -> Multiport Switch/1
  Constant2/1 -> Multiport Switch/3
  Constant1/1 -> Multiport Switch/2

== system controllerComponents/Generate Next Waypoints/Persistent Excitation ==
  iterationNumber : Inport
  Constant : Constant  Value=ctrl.persistentExcitationSwitch
  Gain : Gain  Gain=pi/180
  Gain2 : Gain  Gain=ctrl.azimuthPerturbationAmplitude*pi/180
  Gain3 : Gain  Gain=2*pi/ctrl.azimuthPerturbationPeriod
  Gain4 : Gain  Gain=ctrl.zenithPerturbationAmplitude*pi/180
  Gain5 : Gain  Gain=2*pi/ctrl.zenithPerturbationPeriod
  Multiport Switch : MultiPortSwitch  Inputs=2
  Mux1 : Mux  Inputs=2
  Mux2 : Mux  Inputs=2
  Trigonometric Function : Trigonometry
  Trigonometric Function1 : Trigonometry  Operator=cos
  Uniform Random Number : UniformRandomNumber  Minimum=-ctrl.azimuthPerturbationAmplitude  Maximum=ctrl.azimuthPerturbationAmplitude  Seed=92881
  Uniform Random Number1 : UniformRandomNumber  Minimum=-ctrl.zenithPerturbationAmplitude  Maximum=ctrl.zenithPerturbationAmplitude  Seed=52787
  basisParameterExcitation : Outport
  wires:
  Gain/1 -> Multiport Switch/3
  Uniform Random Number1/1 -> Mux2/2
  Uniform Random Number/1 -> Mux2/1
  Mux2/1 -> Gain/1
  Mux1/1 -> Multiport Switch/2
  Constant/1 -> Multiport Switch/1
  Multiport Switch/1 -> basisParameterExcitation/1
  iterationNumber/1 -> Gain3/1, Gain5/1
  Gain4/1 -> Mux1/2
  Gain5/1 -> Trigonometric Function1/1
  Trigonometric Function/1 -> Gain2/1
  Trigonometric Function1/1 -> Gain4/1
  Gain2/1 -> Mux1/1
  Gain3/1 -> Trigonometric Function/1

== system controllerComponents/Generate Next Waypoints/Trust Region ==
  deltaBasisIn : Inport
  Abs : Abs
  Abs1 : Abs
  Constant : Constant  Value=ctrl.azimuthDistanceLim
  Constant1 : Constant  Value=ctrl.zenithDistanceLim
  Constant2 : Constant
  Divide : Product  Inputs=*/
  Divide1 : Product  Inputs=*/
  Gain : Gain  Gain=pi/180
  Gain1 : Gain  Gain=pi/180
  MinMax : MinMax  Inputs=3
  Product : Product
  Selector : Selector  InputPortWidth=2  IndexOptions=Index vector (dialog)  Indices=1  OutputSizes=1
  Selector1 : Selector  InputPortWidth=2  IndexOptions=Index vector (dialog)  Indices=2  OutputSizes=1
  deltaBasisOut : Outport
  wires:
  deltaBasisIn/1 -> [deltaBasis]
  Product/1 -> deltaBasisOut/1
  MinMax/1 -> Product/2
  [deltaBasis] -> Product/1
  Constant2/1 -> MinMax/1
  Constant1/1 -> Gain1/1
  [deltaBasis] -> Selector1/1
  Selector1/1 -> Abs1/1
  Selector/1 -> Abs/1
  Divide1/1 -> MinMax/3
  Abs/1 -> Divide/2
  Divide/1 -> MinMax/2
  Constant/1 -> Gain/1
  [deltaBasis] -> Selector/1
  Abs1/1 -> Divide1/2
  Gain/1 -> Divide/1
  Gain1/1 -> Divide1/1

== system controllerComponents/Get Target Point/Select Target Point ==
  closestPointIndex : Inport
  Add : Sum
  Constant : Constant  Value=ctrl.waypointAngles
  Constant1 : Constant  Value=ctrl.lookAheadIndexOffset
  Constant2 : Constant  Value=ctrl.waypointAngles
  Selector1 : Selector  InputPortWidth=ctrl.num  IndexOptions=Index vector (port)  Indices=3  OutputSizes=1
  Selector2 : Selector  InputPortWidth=ctrl.num  IndexOptions=Index vector (port)  Indices=3  OutputSizes=1
  Wrap Index1 : controllerComponents/Wrap Index
  targetWaypointAngle : Outport
  targetWaypointIndex : Outport  Port=2
  closestWaypointAngle : Outport  Port=3
  wires:
  Constant/1 -> Selector1/1
  Constant1/1 -> Add/2
  Selector1/1 -> targetWaypointAngle/1
  Add/1 -> Wrap Index1/1
  Wrap Index1/1 -> targetWaypointIndex/1, Selector1/2  "targetedWaypointIndex"
  closestPointIndex/1 -> [closestPointIndex]
  [closestPointIndex] -> Add/1
  Constant2/1 -> Selector2/1
  [closestPointIndex] -> Selector2/2
  Selector2/1 -> closestWaypointAngle/1

== system controllerComponents/Rudder Controller/Gamma ==
  vApp : Inport
  alphaRudder : Inport  Port=2
  Calculate Rotational Inertia : lowLevel/Calculate Rotational Inertia
  Constant : Constant  Value=1/2
  Constant1 : Constant  Value=env.rho
  Constant2 : Constant  Value=plant.rudderTable.kl1
  Constant3 : Constant  Value=plant.momentArm
  Constant4 : Constant
  Constant5 : Constant  Value=plant.refAreaRudder
  Divide : Product  Inputs=*/
  Dot Product : DotProduct  InputSameDT=on  OutDataTypeStr=Inherit: Inherit via internal rule
  Product : Product  Inputs=8
  Trigonometric Function : Trigonometry  Operator=cos
  Gamma : Outport
  wires:
  Constant3/1 -> Product/7
  Constant5/1 -> Product/5
  Constant/1 -> Product/1
  Constant2/1 -> Product/6
  Constant1/1 -> Product/3
  Dot Product/1 -> Product/4
  vApp/1 -> Dot Product/2, Dot Product/1
  alphaRudder/1 -> Trigonometric Function/1
  Trigonometric Function/1 -> Product/8
  Product/1 -> Gamma/1
  Divide/1 -> Product/2
  Calculate Rotational Inertia/1 -> Divide/2
  Constant4/1 -> Divide/1

== system controllerComponents/Rudder Controller/Reference Model ==
  note: Reference Model:
      | 1/(tauR*s+1)^2
  In1 : Inport
  Add1 : Sum  Inputs=--+
  Calculate Initial Twist : controllerComponents/Calculate Initial Twist
  Constant : Constant  Value=plant.initialTwistRate
  Gain : Gain  Gain=1/(ctrl.tauR^2)
  Gain1 : Gain  Gain=2*ctrl.tauR
  Integrator : Integrator  InitialConditionSource=external
  Integrator2 : Integrator  InitialConditionSource=external  InitialCondition=plant.initialTwist
  headingDes : Outport
  headingDesDot : Outport  Port=2
  headingDesDDot : Outport  Port=3
  wires:
  Gain/1 -> headingDesDDot/1, Integrator/1  "headingDesDDot"
  Integrator/1 -> Integrator2/1, headingDesDot/1, Gain1/1  "headingDesDot"
  Add1/1 -> Gain/1
  Integrator2/1 -> Add1/2, headingDes/1  "headingDes"
  In1/1 -> Add1/3  "headingSP"
  Gain1/1 -> Add1/1
  Calculate Initial Twist/1 -> Integrator2/2
  Constant/1 -> Integrator/2
